simulink library "library"  (R2021a)
settings: Solver=VariableStepAuto  StartTime=0.0  StopTime=10.0  RelTol=1e-3
values from neighbouring files (symbols this model uses):
  sensors = struct()    [setup.m]
  spacecraft = struct()    [setup.m]
undefined symbols (not defined in the file or in its folder): actuators, constants, control, observer, orbit
libraries: vrlib x14, $bdroot x5, cstblocks x1, simulink_extras x1
(part 2 of 2)

== matlab function library/Attitude determination/Sensors/Sun sensor enabled/Sun sensor/MATLAB Function ==
  data: phi input; A_err output; theta input; psi input
function A_err = error_matrix(phi, theta, psi)

A_err = [cos(psi)*cos(theta), cos(psi)*sin(theta)*sin(phi) + sin(psi)*cos(phi),...
    -cos(psi)*sin(theta)*cos(phi) + sin(psi)*sin(phi);...
    -sin(psi)*cos(theta), -sin(psi)*sin(theta)*sin(phi) + cos(psi)*cos(phi),...
    sin(psi)*sin(theta)*cos(phi) + cos(psi)*sin(phi);...
    sin(theta), -cos(theta)*sin(phi), cos(theta)*cos(phi)];
            
end

== matlab function library/Attitude determination/Sensors/Sun sensor not enabled/Star tracker/MATLAB Function ==
  data: A_bn input; s_b output; phi input; theta input; psi input; v_n_old input; v_n output; sensors parameter
function [s_b, v_n] = starTracker(A_bn, phi, theta, psi, v_n_old, sensors)

A_sb = sensors.st.A_sb;
nStars = sensors.st.nStars;
FoV = sensors.st.FoV;

A_bs = A_sb';
A_ns = A_bn'*A_bs;

% Preallocation
s_b = zeros(3,nStars); 
v_n = zeros(3,nStars);

El = zeros(nStars,1);
Az = zeros(nStars,1);

for k = 0:nStars-1
    
    % Determining the position in the body and sensor frame of the star at
    % the previous time instant
    s_b_old = A_bn*v_n_old(:,end-k);
    v_s_old = A_sb*s_b_old;
    
    % Computing elevation and azimuth
    El_old = asin(v_s_old(3));
    Az_old = acos(v_s_old(1)/cos(El_old));
    
    % The azimuth shall be comprised between -pi and pi
    if v_s_old(2) <= 0
        Az_old = -Az_old;
    end
    
    % If the star is not anymore in the FoV of the sensor, a new star is
    % generated
    if abs(Az_old) > FoV(1) || abs(El_old) > FoV(2)
        Az(end-k) = 0.2*FoV(1)*(-1 + 2*rand(1,1));
        El(end-k) = 0.2*FoV(2)*(-1 + 2*rand(1,1));
        v_s = [cos(El(end-k))*cos(Az(end-k));...
            cos(El(end-k))*sin(Az(end-k));...
            sin(El(end-k))];
    else
        v_s = v_s_old;
    end
    
    % Error matrix
    A_err = [cos(psi)*cos(theta), cos(psi)*sin(theta)*sin(phi) + sin(psi)*cos(phi),...
        -cos(psi)*sin(theta)*cos(phi) + sin(psi)*sin(phi);...
        -sin(psi)*cos(theta), -sin(psi)*sin(theta)*sin(phi) + cos(psi)*cos(phi),...
        sin(psi)*sin(theta)*cos(phi) + cos(psi)*sin(phi);...
        sin(theta), -cos(theta)*sin(phi), cos(theta)*cos(phi)];
   
   % Generating the measurement (sensor and body frame)
   s_s = A_err*v_s;
   s_bTemp = A_bs*s_s;
   
   % Allocating the measurement in the measurements matrix + normalization
   s_b(1:3, end-k) = s_bTemp./norm(s_bTemp); 

   % Allocating the inertial direction in the inertial directions matrix +
   % normalization
   v_nTemp = A_ns*v_s;
   v_n(1:3,end-k) = v_nTemp;
   v_n(1:3, end-k) = v_nTemp./norm(v_nTemp);
   
end

end
